simulink model "Pila"  (Simulink 10.0)
settings: Solver=ode3  StartTime=0.0  StopTime=30  FixedStep=1/6400  MaxStep=0.001  MinStep=0.000005  RelTol=1e-3  EnableMultiTasking=on
StopFcn:
  | ComtradeWrite5( RDRE1_UIabc, RDRE1_ANames, RDRE1_Dsignals, RDRE1_DNames, RDRE1_ADCscale, RDRE1_PromtFile, RDRE1_NumFile, RDRE1_FileFormat, RDRE1_TestNum);
  | clear RDRE1_UIabc RDRE1_ANames RDRE1_Dsignals RDRE1_DNames RDRE1_ADCscale  RDRE1_PromtFile RDRE1_NumFile RDRE1_FileFormat RDRE1_TestNum
libraries: simulink x3
settings Model: Creator=ivanovsn  LastModifiedBy=nikonenok
settings DataIOCC: LimitDataPoints=on  SignalLoggingSaveFormat=ModelDataLogs
settings OptimizationCC: ExpressionDepthLimit=2147483647
settings DebuggingCC: SolverPrmCheckMsg=warning  FcnCallInpInsideContextMsg=warning  StateNameClashWarn=warning
settings GRTTargetCC: GeneratePreprocessorConditionals=Disable all
settings ConfigComp: CovExternalEMLEnable=off
settings SimscapeCC: SimscapeNormalizeSystem=off

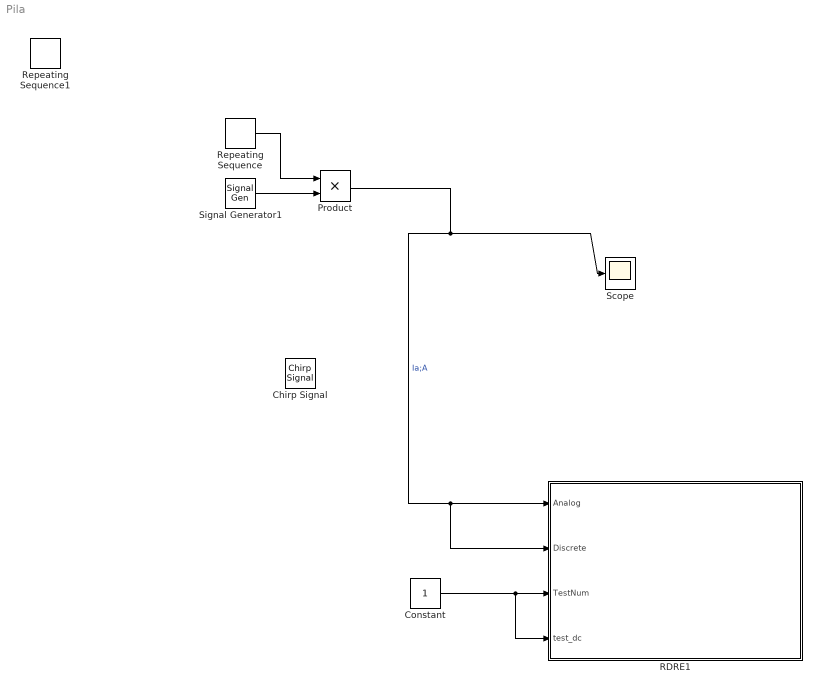
== system Pila ==
  Chirp Signal : simulink/Sources/Chirp Signal  f1=0.1  T=100  f2=1
  Constant : Constant  SampleTime=-1
  Product : Product  RndMeth=Zero
  RDRE1 : Subsystem  mask(RDRE){SamplTime=1/6400, ADCscale=16, FileName=SCADA_test, FileFormat=BINARY}
      mask prompts: SamplTime "Sample time, s"; ADCscale "ADC scale"; FileName "File name"; FileFormat "File format"
      mask help: Сохранение результатов моделирования в формате COMTRADE 1991 (текстовом или бинарном).
      mask init:
      | RDRE_path = gcb;
      | 
      | RDRE_name = get_param (gcb, 'Name');
      | Td = SamplTime;
      | 
      | porthandles = get(gcbh, 'PortHandles');
      | linehandle1 = get(porthandles.Inport(1), 'Line');
      | 
      | if linehandle1 ~= -1
      | set(linehandle1, 'SignalPropagation', 'on');
      | ANames1 = get (porthandles.Inport(1), 'Label');
      | 
      | else ANames1 = 'empty';
      | end
      | 
      | linehandle2 = get(porthandles.Inport(2), 'Line');
      | if linehandle2 ~= -1
      | set(linehandle2, 'SignalPropagation', 'on');
      | DNames1 = get (porthandles.Inport(2), 'Label');
      | 
      | else DNames1 = 'empty';
      | end
      | 
      | 
      | set_param( strcat(RDRE_path, '/' , 'To Workspace'), 'VariableName', 'UIabc' );
      | set_param( strcat(RDRE_path, '/' , 'To Workspace'), 'VariableName', strcat(RDRE_name, '_', 'UIabc'));
      | 
      | set_param( strcat(RDRE_path, '/' , 'To Workspace9'), 'VariableName', 'ANames' );
      | set_param( strcat(RDRE_path, '/' , 'To Workspace9'), 'VariableName', strcat(RDRE_name, '_', 'ANames'));
      | ANames = double (ANames1);
      | 
      | set_param( strcat(RDRE_path, '/' , 'To Workspace1'), 'VariableName', 'ADCscale' );
      | set_param( strcat(RDRE_path, '/' , 'To Workspace1'), 'VariableName', strcat(RDRE_name, '_', 'ADCscale'));
      | 
      | set_param( strcat(RDRE_path, '/' , 'To Workspace11'), 'VariableName', 'PromtFile' );
      | set_param( strcat(RDRE_path, '/' , 'To Workspace11'), 'VariableName', strcat(RDRE_name, '_', 'PromtFile'));
      | % NumPromt = double( PromtFile );
      | 
      | 
      | 
      | set_param( strcat(RDRE_path, '/' , 'To Workspace2'), 'VariableName', 'NumFile' );
      | set_param( strcat(RDRE_path, '/' , 'To Workspace2'), 'VariableName', strcat(RDRE_name, '_', 'NumFile'));
      | NumFile = double( FileName );
      | 
      | set_param( strcat(RDRE_path, '/' , 'To Workspace3'), 'VariableName', 'FileFormat' );
      | set_param( strcat(RDRE_path, '/' , 'To Workspace3'), 'VariableName', strcat(RDRE_name, '_', 'FileFormat'));
      | %FileFormat = double( file_format );
      | 
      | set_param( strcat(RDRE_path, '/' , 'To Workspace4'), 'VariableName', 'Dsignals' );
      | set_param( strcat(RDRE_path, '/' , 'To Workspace4'), 'VariableName', strcat(RDRE_name, '_', 'Dsignals'));
      | 
      | set_param( strcat(RDRE_path, '/' , 'To Workspace10'), 'VariableName', 'DNames' );
      | set_param( strcat(RDRE_path, '/' , 'To Workspace10'), 'VariableName', strcat(RDRE_name, '_', 'DNames'));
      | DNames = double (DNames1);
      | 
      | 
      | Td = SamplTime;
      | 
      | % sys = get_param(bdroot, 'Handle');
      | % l = find_system(sys, 'FindAll', 'on', 'type', 'line')
      | % for i=1:length(l)
      | %       %set(l(i),'signalPropagation','off');
      | %       set(l(i),'signalPropagation','on')
      | % end
      mask Help:
      | Comtrade generator - блок сохранения результатов моделирования в формате COMTRADE
      | (текстовом или бинарном).
      | На входы блока (Analog и Discrete) подаются аналоговые и дискретные сигналы соответственно,
      | объединенные с помощью блоков Mux или Bus Creator.
      | В параметрах блока задаются:
      |  - интервал дискретизации (Sample time);
      |  - разрядность АЦП (ADC scale);
      |  - имя файла осциллограммы (File name);
      |  - заголовок осциллограммы (Promt file);
      |  - формат осциллограммы (File format);
      |  - время записываемого предаварийного режима (Prefault time);
      |  - время записываемого послеаварийного режима (Postfault time);
      |  - длительность записываемой осциллограмы (Limit time);
      |  - Выбор режима записи (Manual). Для выбора РУЧНОГО режима записи
      | необходимо выставить флажок на вкладке MANUAL MODE.
      | В РУЧНОМ режиме осцилограмма записывается с начала (Start time = 0)
      | и ограничивается пользовательским временем симуляции (Stop time)
      | В АВТОМАТИЧЕСКОМ режиме (снять флажок с вкладки MANUAL MODE) осциллограмма ограничивается временами
      | Prefault time, Postfault time, Limit time
      mask TypeOptions FileFormat: ASCII | BINARY
      mask Display: disp( 'WRITE \nCOMTRADE\n\nSNames from labels' )
  Repeating Sequence : simulink/Sources/Repeating Sequence  rep_seq_t=[0 30]  rep_seq_y=[0 1]
  Repeating Sequence1 : simulink/Sources/Repeating Sequence  rep_seq_t=[0 1 2 3 4 5 6 7 8 9 10]  rep_seq_y=[1 0 1 0 1 0 1 0 1 0 1]
  Scope : Scope
  Signal Generator1 : SignalGenerator  Amplitude=1*sqrt(2)  Frequency=50
  wires:
  Signal Generator1/1 -> Product/2
  Product/1 -> Scope/1, RDRE1/1(Analog), RDRE1/2(Discrete)  "Ia;A"
  Constant/1 -> RDRE1/3(TestNum), RDRE1/4(test_dc)
  Repeating Sequence/1 -> Product/1

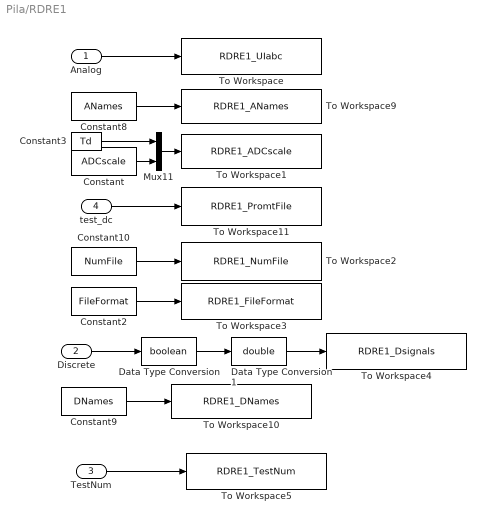
== system Pila/RDRE1 ==
  Analog : Inport
  Discrete : Inport  Port=2
  TestNum : Inport  Port=3
  test_dc : Inport  Port=4
  Constant : Constant  Value=ADCscale
  Constant10 : Constant  Value=NumFile
  Constant2 : Constant  Value=FileFormat
  Constant3 : Constant  Value=Td
  Constant8 : Constant  Value=ANames
  Constant9 : Constant  Value=DNames
  Data Type Conversion : DataTypeConversion  OutDataTypeStr=boolean  RndMeth=Zero
  Data Type Conversion1 : DataTypeConversion  OutDataTypeStr=double  RndMeth=Zero
  Mux11 : Mux  Inputs=2
  To Workspace : ToWorkspace  VariableName=RDRE1_UIabc  SaveFormat=Structure With Time  SampleTime=Td
  To Workspace1 : ToWorkspace  VariableName=RDRE1_ADCscale  SampleTime=1.e3
  To Workspace10 : ToWorkspace  VariableName=RDRE1_DNames  SampleTime=1.e3
  To Workspace11 : ToWorkspace  VariableName=RDRE1_PromtFile  SampleTime=-1
  To Workspace2 : ToWorkspace  VariableName=RDRE1_NumFile  SampleTime=1.e3
  To Workspace3 : ToWorkspace  VariableName=RDRE1_FileFormat  SampleTime=1.e3
  To Workspace4 : ToWorkspace  VariableName=RDRE1_Dsignals  SaveFormat=Structure With Time  SampleTime=Td
  To Workspace5 : ToWorkspace  VariableName=RDRE1_TestNum  SampleTime=Td
  To Workspace9 : ToWorkspace  VariableName=RDRE1_ANames  SampleTime=1.e3
  wires:
  test_dc/1 -> To Workspace11/1
  Constant10/1 -> To Workspace2/1
  Constant8/1 -> To Workspace9/1
  Constant9/1 -> To Workspace10/1
  Constant2/1 -> To Workspace3/1
  Constant3/1 -> Mux11/1
  Mux11/1 -> To Workspace1/1
  Constant/1 -> Mux11/2
  Discrete/1 -> Data Type Conversion/1
  Data Type Conversion/1 -> Data Type Conversion1/1
  Data Type Conversion1/1 -> To Workspace4/1
  Analog/1 -> To Workspace/1
  TestNum/1 -> To Workspace5/1
